simulink model "MAE275_A7E1_2015"  (Simulink 7.7)
settings: Solver=ode45  StartTime=0.0  StopTime=25  RelTol=1e-3
values from neighbouring files (symbols this model uses):
  A = [X_u + a * X_wdot * Z_u   X_w + a * X_wdot * Z_w   X_q + a * X_wdot * (u_0 + Z_q)   -g * (cos(theta_0) + a * X_wdot * sin(theta_0)) 0 ... (first row only)    [f.m]
  B = [a * X_wdot * Z_d_e + X_d_e  a * X_wdot * Z_d_T + X_d_T  -(X_u + a * X_wdot * Z_u)  -(X_w + a * X_wdot * Z_w)  -(X_q + a * X_wdot * (u_0 + Z_q)) ... (first row only)    [f.m]
  C = [1 0 0 0 0 ... (first row only)    [f.m]
  D = [0 0 0 0 0 ... (first row only)    [f.m]
  Kp_h = 0.00173    [f.m]
  Kp_theta = 1.75    [f.m]
libraries: simulink x5
settings Model: Creator=hess  LastModifiedBy=hess

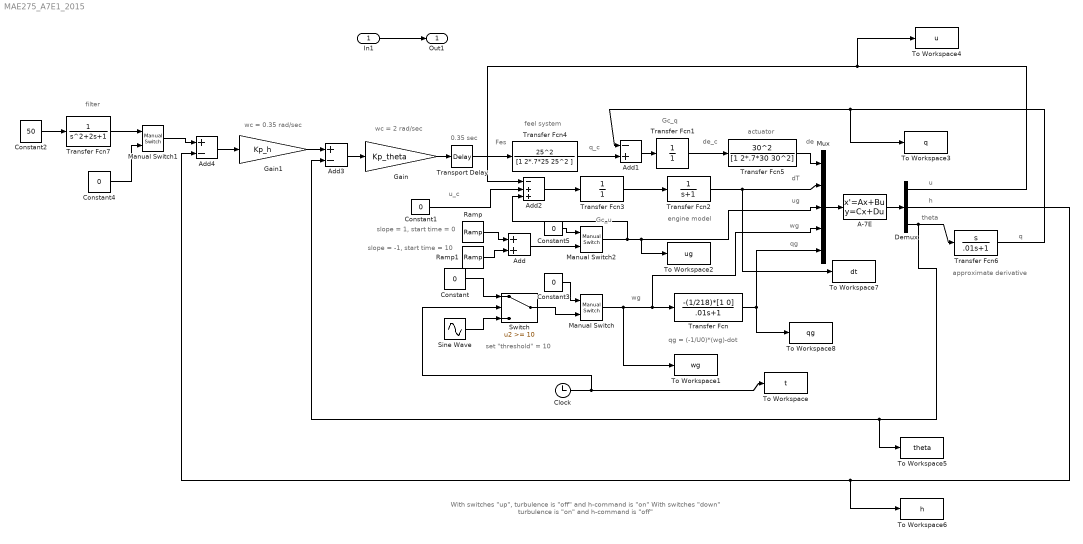
== system MAE275_A7E1_2015 ==
  note: wc = 0.35 rad/sec
  note: wc = 2 rad/sec
  note: Gc_q
  note: Gc_u
  note: 0.35 sec
  note: feel system
  note: engine model
  note: actuator
  note: de
  note: dT
  note: ug
  note: wg
  note: qg
  note: set "threshold" = 10
  note: q
  note: h
  note: theta
  note: u
  note: wg
  note: slope = -1, start time = 10
  note: slope = 1, start time = 0
  note: filter
  note: qg = (-1/U0)*(wg)-dot
  note: de_c
  note: approximate derivative
  note: Fes
  note: q_c
  note: u_c
  note: With switches "up", turbulence is "off" and h-command is "on"
      | With switches "down" turbulence is "on" and h-command is "off"
  In1 : Inport
  A-7E : StateSpace  A=A  B=B  C=C  D=D  X0=[0 0 0 0 0]
  Add : Sum
  Add1 : Sum  Inputs=-+
  Add2 : Sum  Inputs=-++
  Add3 : Sum  Inputs=+-
  Add4 : Sum  Inputs=+-
  Clock : Clock
      settings: Decimation=10
  Constant{,1,3..5} (5 alike) : Constant  Value=0
  Constant2 : Constant  Value=50
  Demux : Demux  Outputs=3
  Gain : Gain  Gain=Kp_theta
  Gain1 : Gain  Gain=Kp_h
  Manual Switch : simulink/Signal Routing/Manual Switch  SystemSampleTime=-1  sw=0  action=0  varsize=off
  Manual Switch1 : simulink/Signal Routing/Manual Switch  SystemSampleTime=-1  sw=0  action=0  varsize=off
  Manual Switch2 : simulink/Signal Routing/Manual Switch  SystemSampleTime=-1  sw=0  action=0  varsize=off
  Mux : Mux  Inputs=5
  Ramp : simulink/Sources/Ramp  SystemSampleTime=-1  slope=1  start=0  X0=0
  Ramp1 : simulink/Sources/Ramp  SystemSampleTime=-1  slope=-1  start=10  X0=0
  Sine Wave : Sin  Amplitude=-5  Frequency=0.2*pi  SampleTime=0
  Switch : Switch  Threshold=10
  To Workspace : ToWorkspace  VariableName=t  SampleTime=-1  SaveFormat=Array
  To Workspace1 : ToWorkspace  VariableName=wg  SampleTime=-1  SaveFormat=Array
  To Workspace2 : ToWorkspace  VariableName=ug  SampleTime=-1  SaveFormat=Array
  To Workspace3 : ToWorkspace  VariableName=q  SampleTime=-1  SaveFormat=Array
  To Workspace4 : ToWorkspace  VariableName=u  SampleTime=-1  SaveFormat=Array
  To Workspace5 : ToWorkspace  VariableName=theta  SampleTime=-1  SaveFormat=Array
  To Workspace6 : ToWorkspace  VariableName=h  SampleTime=-1  SaveFormat=Array
  To Workspace7 : ToWorkspace  VariableName=dt  SampleTime=-1  SaveFormat=Array
  To Workspace8 : ToWorkspace  VariableName=qg  SampleTime=-1  SaveFormat=Array
  Transfer Fcn : TransferFcn  Numerator=-(1/218)*[1 0]  Denominator=[.01 1]
  Transfer Fcn1 : TransferFcn  Numerator=1  Denominator=1
  Transfer Fcn2 : TransferFcn  Numerator=1  Denominator=[1 1]
  Transfer Fcn3 : TransferFcn  Numerator=1  Denominator=1
  Transfer Fcn4 : TransferFcn  Numerator=25^2  Denominator=[1 2*.7*25 25^2 ]
  Transfer Fcn5 : TransferFcn  Numerator=30^2  Denominator=[1 2*.7*30 30^2]
  Transfer Fcn6 : TransferFcn  Numerator=[1 0]  Denominator=[.01 1]
  Transfer Fcn7 : TransferFcn  Numerator=1
  Transport Delay : TransportDelay  DelayTime=.35  PadeOrder=4
  Out1 : Outport
  wires:
  A-7E/1 -> Demux/1
  Mux/1 -> A-7E/1
  Sine Wave/1 -> Switch/3
  Constant/1 -> Switch/1
  Demux/3 -> Add3/2, To Workspace5/1, Transfer Fcn6/1
  Transfer Fcn2/1 -> To Workspace7/1, Mux/2
  Demux/1 -> Add2/1, To Workspace4/1
  Gain/1 -> Transport Delay/1
  Constant1/1 -> Add2/2
  Demux/2 -> To Workspace6/1, Add4/2
  Constant2/1 -> Transfer Fcn7/1
  Add3/1 -> Gain/1
  Gain1/1 -> Add3/1
  Add2/1 -> Transfer Fcn3/1
  Transfer Fcn3/1 -> Transfer Fcn2/1
  Transfer Fcn1/1 -> Transfer Fcn5/1
  Add1/1 -> Transfer Fcn1/1
  Transfer Fcn4/1 -> Add1/2
  Transfer Fcn6/1 -> To Workspace3/1, Add1/1
  Add4/1 -> Gain1/1
  Transfer Fcn/1 -> Mux/5, To Workspace8/1
  In1/1 -> Out1/1
  Manual Switch/1 -> Transfer Fcn/1, Mux/4, To Workspace1/1
  Manual Switch1/1 -> Add4/1
  Constant4/1 -> Manual Switch1/2
  Transfer Fcn5/1 -> Mux/1
  Ramp/1 -> Add/1
  Transport Delay/1 -> Transfer Fcn4/1
  Clock/1 -> To Workspace/1, Switch/2
  Ramp1/1 -> Add/2
  Add/1 -> Manual Switch2/2
  Manual Switch2/1 -> Add2/3, Mux/3, To Workspace2/1
  Constant5/1 -> Manual Switch2/1
  Constant3/1 -> Manual Switch/1
  Switch/1 -> Manual Switch/2
  Transfer Fcn7/1 -> Manual Switch1/1
